simulink model "primer06_2012"  (R2016b)
settings: Solver=VariableStepAuto  StartTime=0.0  StopTime=10.0  MaxStep=0.01  RelTol=1e-3  EnableMultiTasking=on
values from neighbouring files (symbols this model uses):
  k = 9    [primer06_konstante.m]
  T = 0.1    [Zadatak1_konstatnte.m]    (also in primer01_konstante.m = 1; primer06_konstante.m)
settings Model: Creator=Moon Raven  LastModifiedBy=User
settings OptimizationCC: LifeSpan=inf
settings DebuggingCC: SFUnexpectedBacktrackingDiag=warning  SFNoUnconditionalDefaultTransitionDiag=warning  SFExecutionAtInitializationDiag=none
settings GRTTargetCC: TargetLangStandard=C89/C90 (ANSI)  GeneratePreprocessorConditionals=Disable all
settings ConfigComp: CovMetricSettings=dw  CovHtmlReporting=on  CovSaveCumulativeToWorkspaceVar=on  CovSaveSingleToWorkspaceVar=on  CovExternalEMLEnable=off

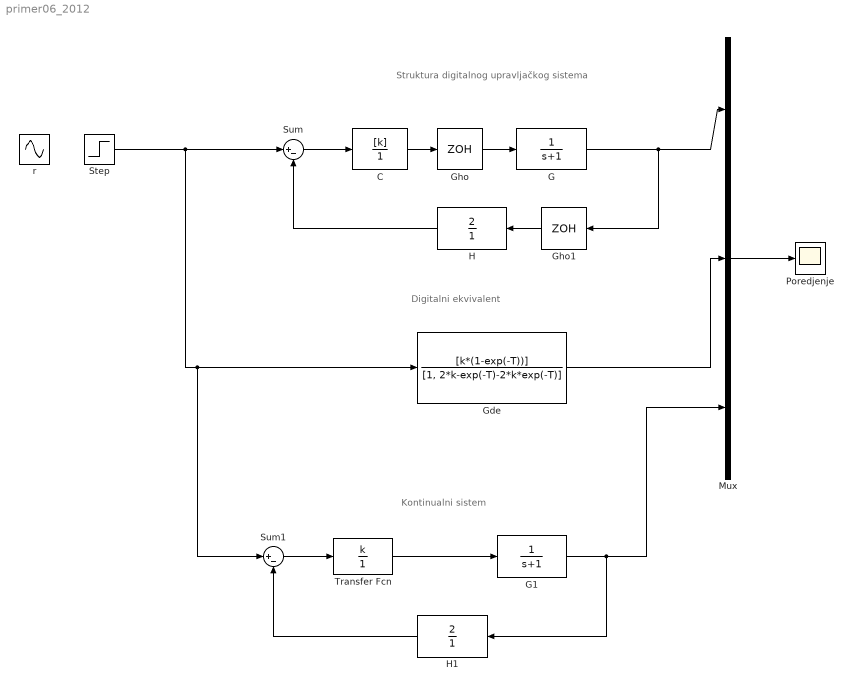
== system primer06_2012 ==
  note: Struktura digitalnog upravljačkog sistema
  note: Digitalni ekvivalent
  note: Kontinualni sistem
  C : DiscreteTransferFcn  Numerator=[k]  Denominator=[1]  SampleTime=T
  G : TransferFcn  Denominator=[1 1]
  G1 : TransferFcn  Denominator=[1 1]
  Gde : DiscreteTransferFcn  Numerator=[k*(1-exp(-T))]  Denominator=[1, 2*k-exp(-T)-2*k*exp(-T)]  SampleTime=T
  Gho : ZeroOrderHold  SampleTime=T
  Gho1 : ZeroOrderHold  SampleTime=T
  H : TransferFcn  Numerator=[2]  Denominator=[1]
  H1 : TransferFcn  Numerator=[2]  Denominator=[1]
  Mux : Mux  Inputs=3
  Poredjenje : Scope
  Step : Step  SampleTime=0
  Sum : Sum  Inputs=|+-
  Sum1 : Sum  Inputs=|+-
  Transfer Fcn : TransferFcn  Numerator=k  Denominator=[1]
  r : Sin  Frequency=0.5  SampleTime=0
  wires:
  Sum/1 -> C/1
  C/1 -> Gho/1
  Gho/1 -> G/1
  G/1 -> Gho1/1, Mux/1
  Gho1/1 -> H/1
  H/1 -> Sum/2
  Gde/1 -> Mux/2
  Mux/1 -> Poredjenje/1
  Sum1/1 -> Transfer Fcn/1
  H1/1 -> Sum1/2
  G1/1 -> H1/1, Mux/3
  Step/1 -> Sum1/1, Gde/1, Sum/1
  Transfer Fcn/1 -> G1/1
